simulink model "SimulinkNews"  (R2025a)
settings: Solver=VariableStepAuto  StartTime=0.0  StopTime=10.0  RelTol=1e-3
libraries: uavalgslib x2, aerolibobsolete x1, simulink x1, uavutilslib x1
settings Model: Creator=Nguyen_Duc  LastModifiedBy=Admin

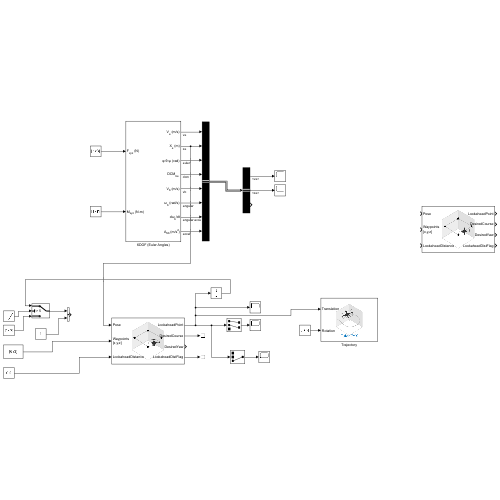
[thumbnail: Simulink's stored preview of the top-level diagram]
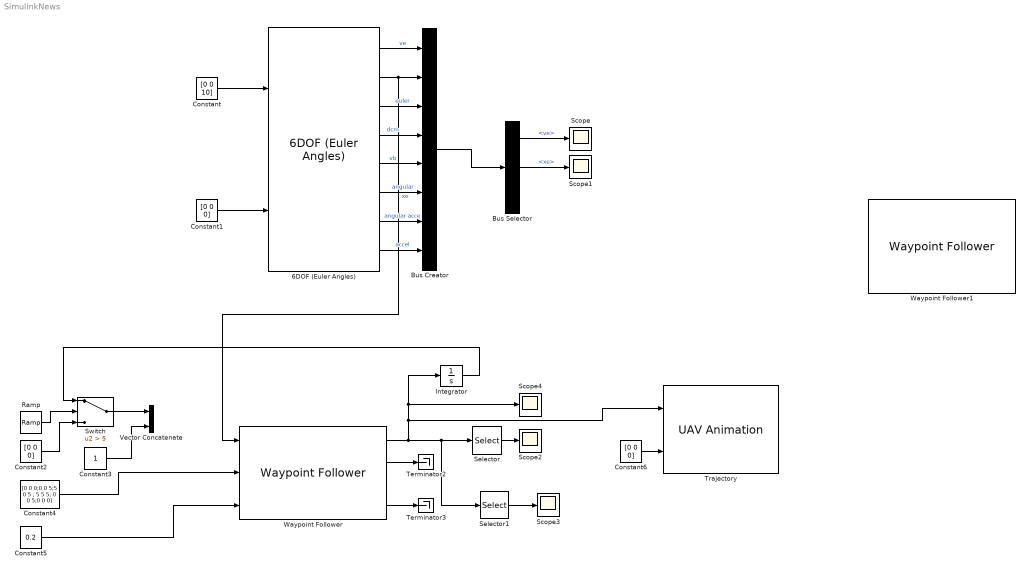
== system SimulinkNews ==
  6DOF (Euler Angles) : aerolibobsolete/6DOF (Euler Angles)  units=Metric (MKS)  mtype=Fixed  rep=Euler Angles  xme_0=[0 0 0]  Vm_0=[0 0 0]  eul_0=[0 0 0]  pm_0=[0 0 0]  mass_0=13  mass_e=0.5  mass_f=2.0  inertia=[0.49827 0 0; 0 0.48993 0; 0 0 0.82777]  inertia_e=eye(3)  inertia_f=2*eye(3)  k_quat=1.0  vre_flag=on  abi_flag=off  aMode=0  xme_statename=''  Vm_statename=''  eul_statename=''  quat_statename=''  pm_statename=''  mass_statename=''
  Bus Creator : BusCreator  Inputs=8
  Bus Selector : BusSelector  OutputSignals=ve,xe,euler
  Constant : Constant  Value=[0 0 10]
  Constant1 : Constant  Value=[0 0 0]
  Constant2 : Constant  Value=[0 0 0]
  Constant3 : Constant
  Constant4 : Constant  Value=[0 0 0;0 0 5;5 0 5 ; 5 5 5; 0 0 5;0 0 0]  VectorParams1D=off
  Constant5 : Constant  Value=0.2
  Constant6 : Constant  Value=[0 0 0]
  Integrator : Integrator
  Ramp : simulink/Sources/Ramp  slope=10  start=0  InitialOutput=0
  Scope{,1..4} (5 alike) : Scope
      Scope settings: ActiveDisplayYMinimum=-23.874097781147192  ActiveDisplayYMaximum=13.437901197446275
      Scope1 settings: ActiveDisplayYMinimum=-79.38442295239858  ActiveDisplayYMaximum=35.220268291132435
      Scope2 settings: ActiveDisplayYMinimum=-3.6085820469695582  ActiveDisplayYMaximum=5.9948783376593617  DataLoggingVariableName=ScopeData2
      Scope3 settings: ActiveDisplayYMinimum=-15.990867176983059  ActiveDisplayYMaximum=12.101758261496295  DataLoggingVariableName=ScopeData3
      Scope4 settings: ActiveDisplayYMinimum=-13.503128760716363  ActiveDisplayYMaximum=10.76433733450388  DataLoggingVariableName=ScopeData4
  Selector : Selector  InputPortWidth=3  IndexOptions=Index vector (dialog)  Indices=[1 2]  OutputSizes=1
  Selector1 : Selector  InputPortWidth=3  IndexOptions=Index vector (dialog)  Indices=[3]  OutputSizes=1
  Switch : Switch  Criteria=u2 > Threshold  Threshold=5  SaturateOnIntegerOverflow=off  InputSameDT=off
  Terminator2 : Terminator
  Terminator3 : Terminator
  Trajectory : uavutilslib/UAV Animation  NumUAV=1  DynamicUAVConfig=off  UAVType=Multirotor  UAVSize=5  UAVColor=[1 0 0]  UAVTrajectoryAlpha=1  InertialZDirection=Down  RotationFormat=Euler ZYX  DrawMarkers=off  SampleTime=0.1
  Vector Concatenate : Concatenate
  Waypoint Follower : uavalgslib/Waypoint Follower  UAVType=multirotor  StartFrom=first  TransitionRadiusSource=internal  TransitionRadius=10  MinLookaheadDistance=0.1  HoverAtLastWaypoint=off  YawInput=off  ShowCrossTrackErrorOutput=off  ShowStatusOutput=off  SimulateUsing=Interpreted execution
  Waypoint Follower1 : uavalgslib/Waypoint Follower  UAVType=multirotor  StartFrom=first  TransitionRadiusSource=internal  TransitionRadius=10  MinLookaheadDistance=0.1  HoverAtLastWaypoint=off  YawInput=off  ShowCrossTrackErrorOutput=off  ShowStatusOutput=off  SimulateUsing=Interpreted execution
  wires:
  Constant/1 -> 6DOF (Euler Angles)/1
  Constant1/1 -> 6DOF (Euler Angles)/2
  6DOF (Euler Angles)/1 -> Bus Creator/1  "ve"
  6DOF (Euler Angles)/2 -> Waypoint Follower/1, Bus Creator/2  "xe"
  6DOF (Euler Angles)/3 -> Bus Creator/3  "euler"
  6DOF (Euler Angles)/4 -> Bus Creator/4  "dcm"
  6DOF (Euler Angles)/5 -> Bus Creator/5  "vb"
  6DOF (Euler Angles)/6 -> Bus Creator/6  "angular"
  6DOF (Euler Angles)/7 -> Bus Creator/7  "angular acce"
  6DOF (Euler Angles)/8 -> Bus Creator/8  "accel"
  Bus Creator/1 -> Bus Selector/1
  Bus Selector/1 -> Scope/1  "<ve>"
  Bus Selector/2 -> Scope1/1  "<xe>"
  Waypoint Follower/2 -> Terminator2/1
  Ramp/1 -> Switch/2
  Constant3/1 -> Vector Concatenate/2
  Constant4/1 -> Waypoint Follower/2
  Waypoint Follower/4 -> Terminator3/1
  Constant2/1 -> Switch/3
  Constant5/1 -> Waypoint Follower/3
  Integrator/1 -> Switch/1
  Switch/1 -> Vector Concatenate/1
  Selector/1 -> Scope2/1
  Selector1/1 -> Scope3/1
  Waypoint Follower/1 -> Trajectory/1, Scope4/1, Integrator/1, Selector1/1, Selector/1
  Constant6/1 -> Trajectory/2
